simulink model "BLOC_gearbox_and_differential"  (R2016a)
settings: Solver=VariableStepAuto  StartTime=0.0  StopTime=10.0  RelTol=1e-3
undefined symbols (not defined in the file): fa_differential_ratio, fa_gearbox_efficiency, fa_gearbox_ratio, hev_dt
settings Model: Creator=Florent  LastModifiedBy=Florent
settings OptimizationCC: DefaultParameterBehavior=Inlined  OptimizeModelRefInitCode=on  LifeSpan=1
settings RTWCC: SystemTargetFile=ert.tlc  TemplateMakefile=ert_default_tmf  GenerateReport=on  IncludeHyperlinkInReport=on  LaunchReport=on  TargetLang=C++  GenerateTraceInfo=on  GenerateTraceReport=on  GenerateTraceReportSl=on  GenerateTraceReportSf=on  GenerateTraceReportEml=on
settings CodeAppCC: ForceParamTrailComments=on  OperatorAnnotations=on  SimulinkDataObjDesc=on  SFDataObjDesc=on  MATLABFcnDesc=on  InsertBlockDesc=on  MATLABSourceComments=on
settings ERTTargetCC: GenerateSampleERTMain=on  MultiInstanceERTCode=on  CodeInterfacePackaging=C++ class  InlinedParameterPlacement=NonHierarchical  RootIOFormat=Structure reference  ERTCustomFileTemplate=example_file_process.tlc

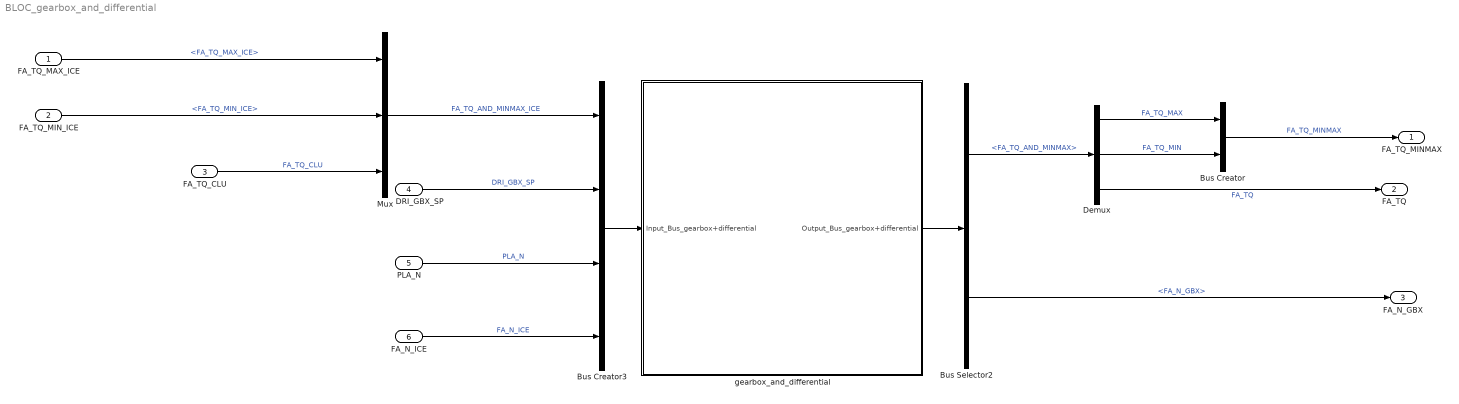
== system BLOC_gearbox_and_differential ==
  FA_TQ_MAX_ICE : Inport
  FA_TQ_MIN_ICE : Inport  Port=2
  FA_TQ_CLU : Inport  Port=3
  DRI_GBX_SP : Inport  Port=4
  PLA_N : Inport  Port=5
  FA_N_ICE : Inport  Port=6
  Bus Creator : BusCreator  Inputs=2
  Bus Creator3 : BusCreator  Inputs=4
  Bus Selector2 : BusSelector  OutputSignals=FA_TQ_AND_MINMAX,FA_N_GBX
  Demux : Demux  Outputs=3
  Mux : Mux  Inputs=3
  gearbox_and_differential : Subsystem  TreatAsAtomicUnit=on  SystemSampleTime=hev_dt
  FA_TQ_MINMAX : Outport  PortDimensions=2
  FA_TQ : Outport  Port=2
  FA_N_GBX : Outport  Port=3
  wires:
  Bus Creator/1 -> FA_TQ_MINMAX/1  "FA_TQ_MINMAX"
  Bus Selector2/1 -> Demux/1  "<FA_TQ_AND_MINMAX>"
  Demux/1 -> Bus Creator/1  "FA_TQ_MAX"
  Demux/2 -> Bus Creator/2  "FA_TQ_MIN"
  Demux/3 -> FA_TQ/1  "FA_TQ"
  FA_TQ_CLU/1 -> Mux/3  "FA_TQ_CLU"
  gearbox_and_differential/1(Output_Bus_gearbox+differential) -> Bus Selector2/1
  Bus Selector2/2 -> FA_N_GBX/1  "<FA_N_GBX>"
  Mux/1 -> Bus Creator3/1  "FA_TQ_AND_MINMAX_ICE"
  DRI_GBX_SP/1 -> Bus Creator3/2  "DRI_GBX_SP"
  PLA_N/1 -> Bus Creator3/3  "PLA_N"
  FA_N_ICE/1 -> Bus Creator3/4  "FA_N_ICE"
  Bus Creator3/1 -> gearbox_and_differential/1(Input_Bus_gearbox+differential)
  FA_TQ_MAX_ICE/1 -> Mux/1  "<FA_TQ_MAX_ICE>"
  FA_TQ_MIN_ICE/1 -> Mux/2  "<FA_TQ_MIN_ICE>"

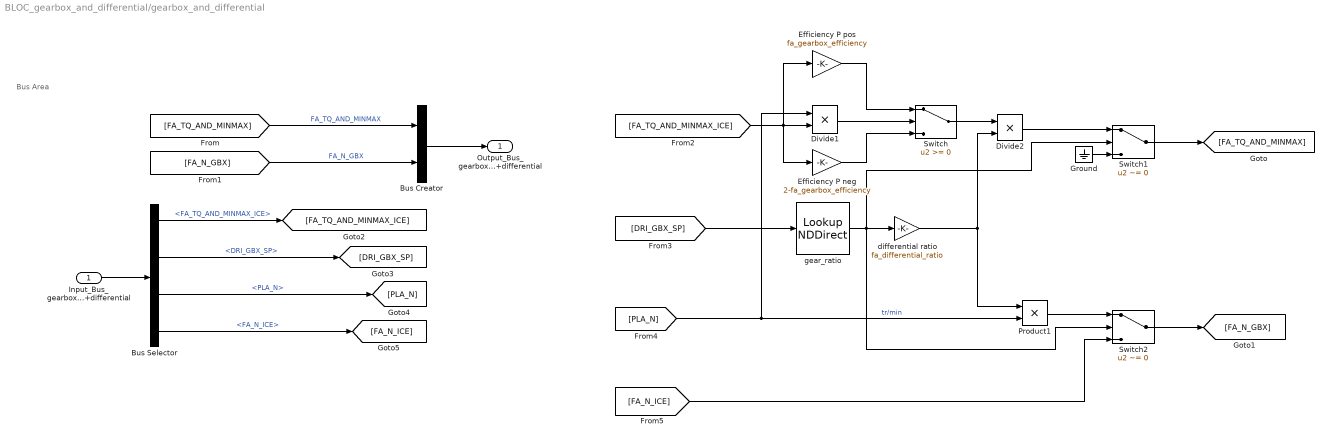
== system BLOC_gearbox_and_differential/gearbox_and_differential ==
  note: Bus Area
  Input_Bus_gearbox+differential : Inport
  " gear_ratio" : LookupNDDirect  NumberOfTableDimensions=1  Table=fa_gearbox_ratio  SampleTime=hev_dt
  Bus Creator : BusCreator  Inputs=2
  Bus Selector : BusSelector  OutputSignals=FA_TQ_AND_MINMAX_ICE,DRI_GBX_SP,PLA_N,FA_N_ICE
  Divide1 : Product  SampleTime=hev_dt
  Divide2 : Product  Inputs=**  SampleTime=hev_dt
  Efficiency P neg : Gain  Gain=2-fa_gearbox_efficiency  SampleTime=hev_dt
  Efficiency P pos : Gain  Gain=fa_gearbox_efficiency  SampleTime=hev_dt
  Ground : Ground
  Product1 : Product  SampleTime=hev_dt  RndMeth=Zero
  Switch : Switch  SampleTime=hev_dt
  Switch1 : Switch  Criteria=u2 ~= 0  SampleTime=hev_dt
  Switch2 : Switch  Criteria=u2 ~= 0  SampleTime=hev_dt
  differential ratio : Gain  Gain=fa_differential_ratio  SampleTime=hev_dt
  Output_Bus_gearbox+differential : Outport
  wires:
  [DRI_GBX_SP] -> " gear_ratio"/1
  " gear_ratio"/1 -> Switch1/2, differential ratio/1, Switch2/2
  differential ratio/1 -> Divide2/2, Product1/1
  Divide2/1 -> Switch1/1
  [FA_TQ_AND_MINMAX_ICE] -> Divide1/2, Efficiency P neg/1, Efficiency P pos/1
  Efficiency P pos/1 -> Switch/1
  Efficiency P neg/1 -> Switch/3
  Divide1/1 -> Switch/2
  Switch/1 -> Divide2/1
  Product1/1 -> Switch2/1
  [PLA_N] -> Product1/2, Divide1/1  "tr/min"
  Switch1/1 -> [FA_TQ_AND_MINMAX]
  Ground/1 -> Switch1/3
  Switch2/1 -> [FA_N_GBX]
  [FA_N_ICE] -> Switch2/3
  Bus Creator/1 -> Output_Bus_gearbox+differential/1
  [FA_TQ_AND_MINMAX] -> Bus Creator/1  "FA_TQ_AND_MINMAX"
  [FA_N_GBX] -> Bus Creator/2  "FA_N_GBX"
  Input_Bus_gearbox+differential/1 -> Bus Selector/1
  Bus Selector/1 -> [FA_TQ_AND_MINMAX_ICE]  "<FA_TQ_AND_MINMAX_ICE>"
  Bus Selector/2 -> [DRI_GBX_SP]  "<DRI_GBX_SP>"
  Bus Selector/3 -> [PLA_N]  "<PLA_N>"
  Bus Selector/4 -> [FA_N_ICE]  "<FA_N_ICE>"
